simulink model "VehicleBody6DOF"  (R2026b)
settings: Solver=VariableStepAuto
undefined symbols (not defined in the file): BdyFrm, EnvGrvty, InertFrm, PlntVehDstCGFrntAxl, PlntVehDstCGRearAxl, PlntVehFrntUnsprgMass, PlntVehInitLatPos, PlntVehInitLatVel, PlntVehInitLongPos, PlntVehInitLongVel, PlntVehInitPitchAng, PlntVehInitPitchRate, PlntVehInitRollAng, PlntVehInitRollRate, PlntVehInitVertPos, PlntVehInitVertVel, PlntVehInitYawAng, PlntVehInitYawRate, PlntVehMass, PlntVehPitchMomentInertia, PlntVehRearUnsprgMass, PlntVehRollMomentInertia, PlntVehTrckWdth, PlntVehYawMomentInertia
libraries: shared6dof x2, autolibutils x1, sharedtransform x1, vehdynlibeom x1
settings Model: ModifiedByFormat=The MathWorks, Inc.  Creator=The MathWorks, Inc.  LastModifiedBy=The MathWorks, Inc.
settings OptimizationCC: ReuseModelBlockBuffer=off

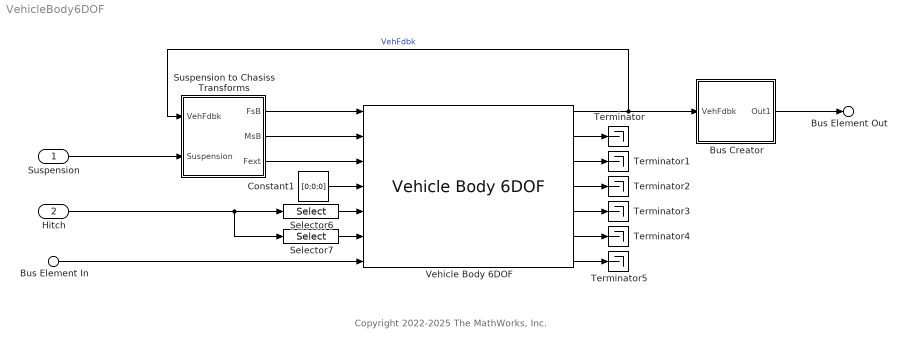
== system VehicleBody6DOF ==
  note: Copyright 2022-2025 The MathWorks, Inc.
  Suspension : Inport
  Hitch : Inport  Port=2
  Bus Element In : Inport  Port=3  PortName=Env  Element=Wind
  Bus Creator : Subsystem
  Constant1 : Constant  Value=[0;0;0]  SampleTime=-1
  Selector6 : Selector  InputPortWidth=6  IndexOptions=Index vector (dialog)  Indices=[1 2 3]  OutputSizes=1
  Selector7 : Selector  InputPortWidth=6  IndexOptions=Index vector (dialog)  Indices=[4 5 6]  OutputSizes=1
  Suspension to Chasiss Transforms : Subsystem
  Terminator{,1..5} (6 alike) : Terminator
  Vehicle Body 6DOF : vehdynlibeom/Vehicle Body 6DOF  extPos=on  extVel=on  extEuler=on  extRotRate=on  htchFMode=on  htchMMode=on  m=PlntVehMass  a=PlntVehDstCGFrntAxl  b=PlntVehDstCGRearAxl  d=0  h=PlntVehCGHgtAxl  dh=PlntVehHtchDst  hl=0  hh=PlntVehHtchHgtAxl  Xe_o=[PlntVehInitLongPos, PlntVehInitLatPos, PlntVehInitVertPos]  xbdot_o=[PlntVehInitLongVel, PlntVehInitLatVel, PlntVehInitVertVel]  eul_o=[PlntVehInitRollAng, PlntVehInitPitchAng, PlntVehInitYawAng]  p_o=[PlntVehInitRollRate, PlntVehInitPitchRate, PlntVehInitYawRate]  Iveh=[PlntVehRollMomentInertia 0 0; 0 PlntVehPitchMomentInertia 0; 0 0 PlntVehYawMomentInertia]  w=PlntVehTrckWdth  z1m=0  z1R=[-.25,.125,.15]  z1I=[1.4,-.2,.1;-.2,1.4,.1;.1,.1,2.25].*0  z2m=0  z2R=[1.4,0,.8]  z2I=[1.4,-.2,.1;-.2,1.4,.1;.1,.1,2.25].*0  z3m=0  z3R=[.75,-.5,.4]  z3I=[5,-.1,-2;-2,9,.1;-.1,.1,6].*0  z4m=0  z4R=[.75,.5,.4]  z4I=[5,-.1,-2;-2,9,.1;-.1,.1,6].*0  z5m=0  z5R=[1.25,-.5,.4]  z5I=[5,-.1,-2;-2,9,.1;-.1,.1,6].*0  z6m=0  z6R=[1.25,-.5,.4]  z6I=[5,-.1,-2;-2,9,.1;-.1,.1,6].*0  z7m=0  z7R=[2,0,.25]  z7I=[1.4,-.2,.1;-.2,1.4,.1;.1,.1,2.25].*0  Af=PlntVehAeroFrntArea  Cd=PlntVehAeroDragCff  Cl=PlntVehAeroLiftCff  Cpm=PlntVehAeroPitchCff  beta_w=PlntVehAeroBetaWindAng  Cs=PlntVehAeroSideCs  Cym=PlntVehAeroYawCym  Pabs=EnvAbsPrs  extTamb=off  Tair=EnvAirTemp  g=EnvGrvty  xdot_tol=.1  longOff=0  latOff=0  vertOff=0.0112  wrapAng=off  aMode=2
  Bus Element Out : Outport  PortName=VehBody
  wires:
  Selector6/1 -> Vehicle Body 6DOF/5
  Selector7/1 -> Vehicle Body 6DOF/6
  Suspension/1 -> Suspension to Chasiss Transforms/2(Suspension)
  Vehicle Body 6DOF/6 -> Terminator4/1
  Vehicle Body 6DOF/7 -> Terminator5/1
  Vehicle Body 6DOF/4 -> Terminator2/1
  Constant1/1 -> Vehicle Body 6DOF/4
  Vehicle Body 6DOF/3 -> Terminator1/1
  Vehicle Body 6DOF/5 -> Terminator3/1
  Vehicle Body 6DOF/2 -> Terminator/1
  Vehicle Body 6DOF/1 -> Bus Creator/1(VehFdbk), Suspension to Chasiss Transforms/1(VehFdbk)  "VehFdbk"
  Bus Element In/1 -> Vehicle Body 6DOF/7
  Hitch/1 -> Selector6/1, Selector7/1
  Suspension to Chasiss Transforms/3(Fext) -> Vehicle Body 6DOF/3
  Suspension to Chasiss Transforms/2(MsB) -> Vehicle Body 6DOF/2
  Suspension to Chasiss Transforms/1(FsB) -> Vehicle Body 6DOF/1
  Bus Creator/1(Out1) -> Bus Element Out/1

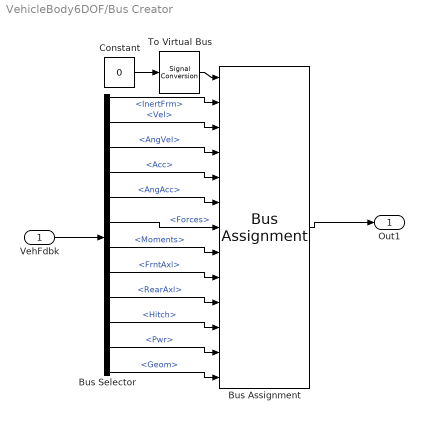
== system VehicleBody6DOF/Bus Creator ==
  VehFdbk : Inport
  Bus Assignment : BusAssignment  AssignedSignals=InertFrm,BdyFrm.Cg.Vel,BdyFrm.Cg.AngVel,BdyFrm.Cg.Acc,BdyFrm.Cg.AngAcc,BdyFrm.Forces,BdyFrm.Moments,BdyFrm.FrntAxl,BdyFrm.RearAxl,BdyFrm.Hitch,BdyFrm.Pwr,BdyFrm.Geom
  Bus Selector : BusSelector  OutputSignals=InertFrm,BdyFrm.Cg.Vel,BdyFrm.Cg.AngVel,BdyFrm.Cg.Acc,BdyFrm.Cg.AngAcc,BdyFrm.Forces,BdyFrm.Moments,BdyFrm.FrntAxl,BdyFrm.RearAxl,BdyFrm.Hitch,BdyFrm.Pwr,BdyFrm.Geom
  Constant : Constant  Value=0  OutDataTypeStr=Bus: VehBodyBUS  SampleTime=Inf
  To Virtual Bus : SignalConversion  ConversionOutput=Virtual bus  OverrideOpt=off
  Out1 : Outport
  wires:
  Bus Assignment/1 -> Out1/1
  Bus Selector/4 -> Bus Assignment/5  "<Acc>"
  Bus Selector/8 -> Bus Assignment/9  "<FrntAxl>"
  Bus Selector/5 -> Bus Assignment/6  "<AngAcc>"
  Bus Selector/12 -> Bus Assignment/13  "<Geom>"
  Bus Selector/3 -> Bus Assignment/4  "<AngVel>"
  Constant/1 -> To Virtual Bus/1
  To Virtual Bus/1 -> Bus Assignment/1
  Bus Selector/1 -> Bus Assignment/2  "<InertFrm>"
  Bus Selector/9 -> Bus Assignment/10  "<RearAxl>"
  Bus Selector/11 -> Bus Assignment/12  "<Pwr>"
  Bus Selector/10 -> Bus Assignment/11  "<Hitch>"
  Bus Selector/7 -> Bus Assignment/8  "<Moments>"
  Bus Selector/2 -> Bus Assignment/3  "<Vel>"
  VehFdbk/1 -> Bus Selector/1
  Bus Selector/6 -> Bus Assignment/7  "<Forces>"

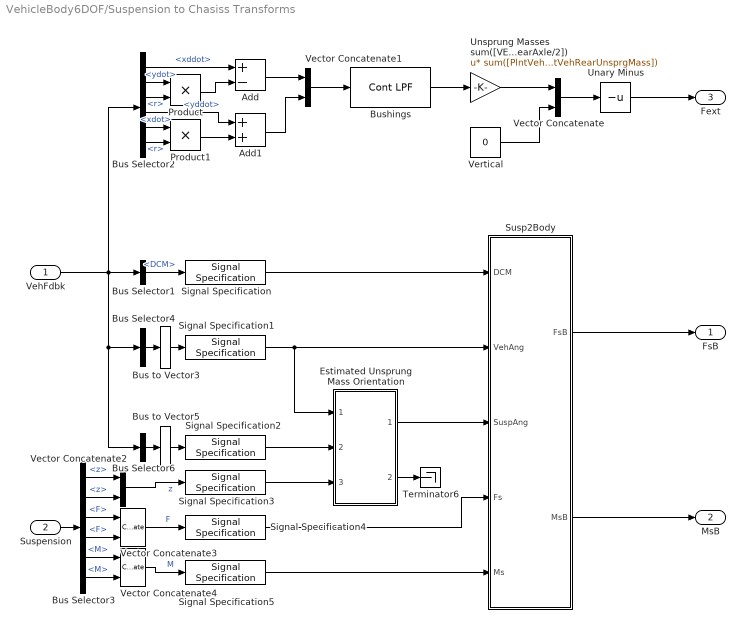
== system VehicleBody6DOF/Suspension to Chasiss Transforms ==
  VehFdbk : Inport
  Suspension : Inport  Port=2
  Add : Sum  Inputs=+-
  Add1 : Sum
  Bus Selector1 : BusSelector  OutputSignals=BdyFrm.Cg.DCM
  Bus Selector2 : BusSelector  OutputSignals=BdyFrm.Cg.Acc.xddot,BdyFrm.Cg.Vel.ydot,BdyFrm.Cg.AngVel.r,BdyFrm.Cg.Acc.yddot,BdyFrm.Cg.Vel.xdot,BdyFrm.Cg.AngVel.r
  Bus Selector3 : BusSelector  OutputSignals=FrntSusp.FrntSuspChassis.Whl.z,RearSusp.RearSuspChassis.Whl.z,FrntSusp.FrntSuspChassis.Veh.F,RearSusp.RearSuspChassis.Veh.F,FrntSusp.FrntSuspChassis.Veh.M,RearSusp.RearSuspChassis.Veh.M
  Bus Selector4 : BusSelector  OutputSignals=InertFrm.Cg.Ang.phi,InertFrm.Cg.Ang.theta,InertFrm.Cg.Ang.psi  OutputAsBus=on
  Bus Selector6 : BusSelector  OutputSignals=InertFrm.Geom.Disp.X,InertFrm.Geom.Disp.Y,InertFrm.Geom.Disp.Z  OutputAsBus=on
  Bus to Vector3 : BusToVector
  Bus to Vector5 : BusToVector
  Bushings : autolibutils/Cont LPF  wc=40*pi.*ones(2,1)  AbsoluteTolerance=auto  aMode=2
  Estimated Unsprung Mass Orientation : MATLAB Function  TreatAsAtomicUnit=on  mask{trackW=PlntVehTrckWdth(1), wheelB=PlntVehDstCGFrntAxl+PlntVehDstCGRearAxl}
      mask prompts: trackW "Vehicle track width, trackW [m]:"; wheelB "Vehicle wheelbase, wheelB [m]:"
      mask help: This block converts wheel ground height information into estimates of vehicle pitch, roll angles and vertical height in order to help in the visualization 3DOF based simulations with changes in terrain. Note that the resulting signals are only used as a visualization aid and do not account for the physical affects of the vehicle interacting with variable terrain or changes in orientation.
  Product : Product
  Product1 : Product
  Signal Specification : SignalSpecification  Dimensions=[3,3]
  Signal Specification1 : SignalSpecification  Dimensions=3
  Signal Specification2 : SignalSpecification  Dimensions=3
  Signal Specification3 : SignalSpecification  Dimensions=4
  Signal Specification4 : SignalSpecification  Dimensions=[3,4]
  Signal Specification5 : SignalSpecification  Dimensions=[3,4]
  Susp2Body : Subsystem
  Terminator6 : Terminator
  Unary Minus : UnaryMinus
  Unsprung Masses sum([VEH.UnsprungMassFrontAxle/2 VEH.UnsprungMassFrontAxle/2 VEH.UnsprungMassRearAxle/2 VEH.UnsprungMassRearAxle/2]) : Gain  Gain=sum([PlntVehFrntUnsprgMass PlntVehRearUnsprgMass])  Multiplication=Matrix(u*K)
  Vector Concatenate : Concatenate
  Vector Concatenate1 : Concatenate
  Vector Concatenate2 : Concatenate
  Vector Concatenate3 : Concatenate  Mode=Multidimensional array  ConcatenateDimension=2
  Vector Concatenate4 : Concatenate  Mode=Multidimensional array  ConcatenateDimension=2
  Vertical : Constant  Value=0  SampleTime=-1
  FsB : Outport  PortDimensions=[3,4]
  MsB : Outport  Port=2  PortDimensions=[3,4]
  Fext : Outport  Port=3  PortDimensions=3
  wires:
  Bus Selector3/5 -> Vector Concatenate4/1  "<M>"
  Bus Selector3/6 -> Vector Concatenate4/2  "<M>"
  Bus Selector3/3 -> Vector Concatenate3/1  "<F>"
  Bus Selector3/4 -> Vector Concatenate3/2  "<F>"
  Bus Selector3/2 -> Vector Concatenate2/2  "<z>"
  Bus Selector3/1 -> Vector Concatenate2/1  "<z>"
  Unary Minus/1 -> Fext/1
  Bus Selector2/1 -> Add/1  "<xddot>"
  Add1/1 -> Vector Concatenate1/2
  Bus Selector2/4 -> Add1/1  "<yddot>"
  Product1/1 -> Add1/2
  Product/1 -> Add/2
  Add/1 -> Vector Concatenate1/1
  Bus Selector2/6 -> Product1/2  "<r>"
  Bus Selector2/5 -> Product1/1  "<xdot>"
  Bus Selector2/3 -> Product/2  "<r>"
  Bus Selector2/2 -> Product/1  "<ydot>"
  Vertical/1 -> Vector Concatenate/2
  Vector Concatenate/1 -> Unary Minus/1
  Susp2Body/1(FsB) -> FsB/1
  Unsprung Masses sum([VEH.UnsprungMassFrontAxle/2 VEH.UnsprungMassFrontAxle/2 VEH.UnsprungMassRearAxle/2 VEH.UnsprungMassRearAxle/2])/1 -> Vector Concatenate/1
  Vector Concatenate1/1 -> Bushings/1
  Bushings/1 -> Unsprung Masses sum([VEH.UnsprungMassFrontAxle/2 VEH.UnsprungMassFrontAxle/2 VEH.UnsprungMassRearAxle/2 VEH.UnsprungMassRearAxle/2])/1
  Susp2Body/2(MsB) -> MsB/1
  Estimated Unsprung Mass Orientation/1(angles) -> Susp2Body/3(SuspAng)
  Vector Concatenate2/1 -> Signal Specification3/1  "z"
  Estimated Unsprung Mass Orientation/2(GeomXYZ) -> Terminator6/1
  Bus Selector4/1 -> Bus to Vector3/1
  Suspension/1 -> Bus Selector3/1
  Bus to Vector5/1 -> Signal Specification2/1
  Bus Selector1/1 -> Signal Specification/1  "<DCM>"
  Bus to Vector3/1 -> Signal Specification1/1
  Vector Concatenate4/1 -> Signal Specification5/1  "M"
  VehFdbk/1 -> Bus Selector4/1, Bus Selector6/1, Bus Selector1/1, Bus Selector2/1
  Vector Concatenate3/1 -> Signal Specification4/1  "F"
  Bus Selector6/1 -> Bus to Vector5/1
  Signal Specification/1 -> Susp2Body/1(DCM)
  Signal Specification1/1 -> Estimated Unsprung Mass Orientation/1(angleIn), Susp2Body/2(VehAng)
  Signal Specification2/1 -> Estimated Unsprung Mass Orientation/2(GemoXYZIn)
  Signal Specification3/1 -> Estimated Unsprung Mass Orientation/3(Ground)
  Signal Specification4/1 -> Susp2Body/4(Fs)
  Signal Specification5/1 -> Susp2Body/5(Ms)

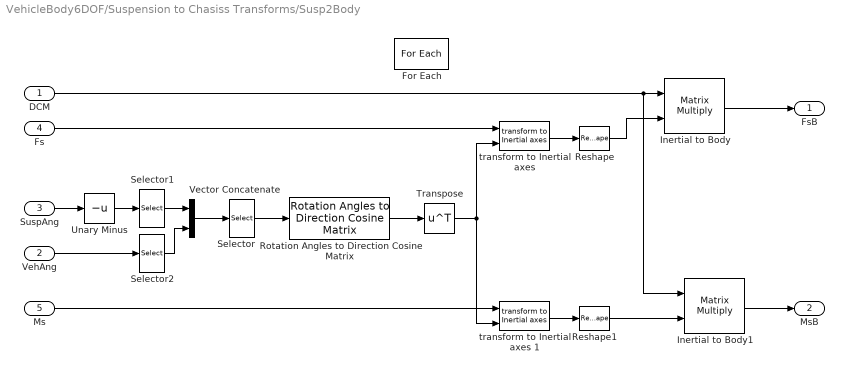
== system VehicleBody6DOF/Suspension to Chasiss Transforms/Susp2Body ==
  DCM : Inport
  VehAng : Inport  Port=2
  SuspAng : Inport  Port=3
  Fs : Inport  Port=4  Partition=on  PartitionDimension=2  PartitionWidth=1  PartitionOffset=0
  Ms : Inport  Port=5  Partition=on  PartitionDimension=2  PartitionWidth=1  PartitionOffset=0
  For Each : ForEach  DisableCoverage=on
  Inertial to Body : Product  Multiplication=Matrix(*)  InputSameDT=on  SaturateOnIntegerOverflow=on  OutDataTypeStr=Inherit: Same as first input
  Inertial to Body1 : Product  Multiplication=Matrix(*)  InputSameDT=on  SaturateOnIntegerOverflow=on  OutDataTypeStr=Inherit: Same as first input
  Reshape : Reshape
  Reshape1 : Reshape
  Rotation Angles to Direction Cosine Matrix : sharedtransform/Rotation Angles to Direction Cosine Matrix  rotationOrder=ZYX  aMode=2
  Selector : Selector  InputPortWidth=3  IndexOptions=Index vector (dialog)  Indices=[3 2 1]  OutputSizes=1
  Selector1 : Selector  InputPortWidth=3  IndexOptions=Index vector (dialog)  Indices=[1 2]  OutputSizes=1
  Selector2 : Selector  InputPortWidth=3  IndexOptions=Index vector (dialog)  Indices=[3]  OutputSizes=1
  Transpose : Math  Operator=transpose  SignedPower=on
  Unary Minus : UnaryMinus
  Vector Concatenate : Concatenate
  "transform to Inertial axes " : shared6dof/6DOF (Euler Angles)/transform to Inertial axes   SystemSampleTime=-1  VariantActivationTime=update diagram  EmptyChoice=off  PassThrough=off  PassThroughVariantControl=(default)  EmptyChoiceVariantControl=(default)  AllowFlexibleInterface=on  Latency=0  AutoFrameSizeCalculation=off
  transform to Inertial axes 1 : shared6dof/6DOF (Euler Angles)/transform to Inertial axes   SystemSampleTime=-1  VariantActivationTime=update diagram  EmptyChoice=off  PassThrough=off  PassThroughVariantControl=(default)  EmptyChoiceVariantControl=(default)  AllowFlexibleInterface=on  Latency=0  AutoFrameSizeCalculation=off
  FsB : Outport  ConcatenationDimension=2  VectorParamsAs1DForOutWhenUnconnected=off
  MsB : Outport  Port=2  ConcatenationDimension=2  VectorParamsAs1DForOutWhenUnconnected=off
  wires:
  Selector2/1 -> Vector Concatenate/2
  Vector Concatenate/1 -> Selector/1
  Selector1/1 -> Vector Concatenate/1
  Unary Minus/1 -> Selector1/1
  VehAng/1 -> Selector2/1
  Ms/1 -> transform to Inertial axes 1/1
  DCM/1 -> Inertial to Body/1, Inertial to Body1/1
  Reshape1/1 -> Inertial to Body1/2
  Inertial to Body1/1 -> MsB/1
  transform to Inertial axes 1/1 -> Reshape1/1
  "transform to Inertial axes "/1 -> Reshape/1
  Rotation Angles to Direction Cosine Matrix/1 -> Transpose/1
  Transpose/1 -> "transform to Inertial axes "/2, transform to Inertial axes 1/2
  Fs/1 -> "transform to Inertial axes "/1
  Selector/1 -> Rotation Angles to Direction Cosine Matrix/1
  SuspAng/1 -> Unary Minus/1
  Inertial to Body/1 -> FsB/1
  Reshape/1 -> Inertial to Body/2

== matlab function VehicleBody6DOF/Suspension to Chasiss Transforms/Estimated Unsprung Mass Orientation ==
  data: angles output size=3; angleIn input size=3; GeomXYZ output size=3; GemoXYZIn input size=3; Ground input size=4; trackW parameter; wheelB parameter
function [angles,GeomXYZ]= three26(angleIn, GemoXYZIn, Ground,trackW, wheelB)%#codegen
coder.allowpcode('plain')
% Copyright 2018 The MathWorks, Inc.
[angles,GeomXYZ]= vdynthree2six(angleIn, GemoXYZIn, Ground,trackW, wheelB);
